simulink model "untitled"  (R2016a)
settings: Solver=VariableStepAuto  StartTime=0.0  StopTime=10  RelTol=1e-3
undefined symbols (not defined in the file): serial
libraries: instrumentlib x3
settings Model: Creator=emanuele  LastModifiedBy=emanuele

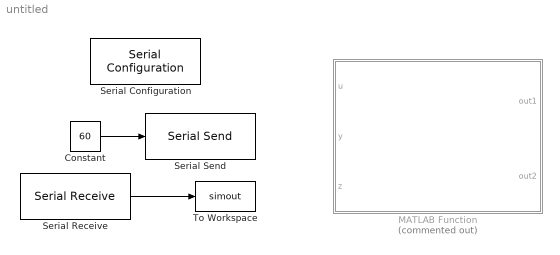
== system untitled ==
  Constant : Constant  Value=60  VectorParams1D=off  OutDataTypeStr=uint8  SampleTime=0.01
  MATLAB Function : MATLAB Function  Commented=on  TreatAsAtomicUnit=on
  Serial Configuration : instrumentlib/Serial Configuration  Priority=-200000  ComPortMenu=/dev/ttyUSB0  ComPort=/dev/ttyUSB0  ObjConstructor=serial('/dev/ttyUSB0');  BaudRate=1000000  DataBits=8  Parity=none  StopBits=1  FlowControl=none  Timeout=10  ByteOrder=LittleEndian
  Serial Receive : instrumentlib/Serial Receive  ComPortMenu=/dev/ttyUSB0  ComPort=/dev/ttyUSB0  ObjConstructor=serial('/dev/ttyUSB0');  Terminator=<none>  DataSize="[1  238]"  DataType=uint8  EnableBlockingMode=on  ActionDataUnavailable=Output last received value  CustomValue=0  SampleTime=0.01
  Serial Send : instrumentlib/Serial Send  ComPortMenu=/dev/ttyUSB0  ComPort=/dev/ttyUSB0  ObjConstructor=serial('/dev/ttyUSB0');  Terminator=<none>  EnableBlockingMode=on
  To Workspace : ToWorkspace  VariableName=simout  SaveFormat=Timeseries  SampleTime=-1
      settings: Save2DSignal=2-D array (concatenate along first dimension)
  wires:
  Constant/1 -> Serial Send/1
  Serial Receive/1 -> To Workspace/1

== matlab function untitled/MATLAB Function ==
  data: u input; out1 output; y input; z input; out2 output
function [out1,out2] = fcn(u,y,z)
%#codegen
    read;
    
    out1 = u * y;
    out2 = z+y;

end
